simulink model "EMGnodev"  (R2016b)
settings: Solver=FixedStepDiscrete  StartTime=0.0  StopTime=Tfinal  FixedStep=0.01  RelTol=1e-3  EnableMultiTasking=on
settings Model: Creator=philipp  LastModifiedBy=anacsousa
settings DataIOCC: LimitDataPoints=on  SaveFormat=Array
settings OptimizationCC: LifeSpan=Inf
settings DebuggingCC: SolverPrmCheckMsg=warning  MultiTaskRateTransMsg=warning  SFUnexpectedBacktrackingDiag=warning  SFNoUnconditionalDefaultTransitionDiag=warning  SFExecutionAtInitializationDiag=none
settings HardwareCC: ProdBitPerPointer=32  ProdBitPerSizeT=32  ProdBitPerPtrDiffT=32  ProdLargestAtomicFloat=None  ProdIntDivRoundTo=Undefined  ProdEndianess=Unspecified  ProdWordSize=32  ProdHWDeviceType=32-bit Generic
settings ModelReferenceCC: PropagateSignalLabelsOutOfModel=off
settings RTWCC: SystemTargetFile=ert_linux.tlc  MakeCommand=make_rtw OPTS=-DWITH_HW  TemplateMakefile=ert_linux.tmf  Description=Linux Embedded Coder  TargetLang=C++
settings CodeAppCC: IgnoreCustomStorageClasses=off
settings STFCustomTargetCC: ModelReferenceCompliant=off  CombineOutputUpdateFcns=on  ERTCustomFileBanners=on  SupportNonInlinedSFcns=off  RemoveResetFunc=on  SupportVariableSizeSignals=on  MATLABClassNameForMDSCustomization=Simulink.SoftwareTarget.ERTCustomization  GRTInterface=off  SystemTargetFile=ert_linux.tlc
settings ERTTargetCC: ModelReferenceCompliant=off  ParMdlRefBuildCompliant=off  CompOptLevelCompliant=off  ConcurrentExecutionCompliant=off  ERTFirstTimeCompliant=off  SupportContinuousTime=on  SupportVariableSizeSignals=on  ModelStepFunctionPrototypeControlCompliant=off  CPPClassGenCompliant=off  UseToolchainInfoCompliant=off  ExtMode=on  ERTCustomFileTemplate=ert_linux_file_process.tlc  ConvertIfToSwitch=off  SuppressUnreachableDefaultCases=off
settings ConfigComp: CovMetricSettings=dw  CovHtmlReporting=on  CovSaveCumulativeToWorkspaceVar=on  CovSaveSingleToWorkspaceVar=on  CovExternalEMLEnable=off  CovSFcnEnable=off

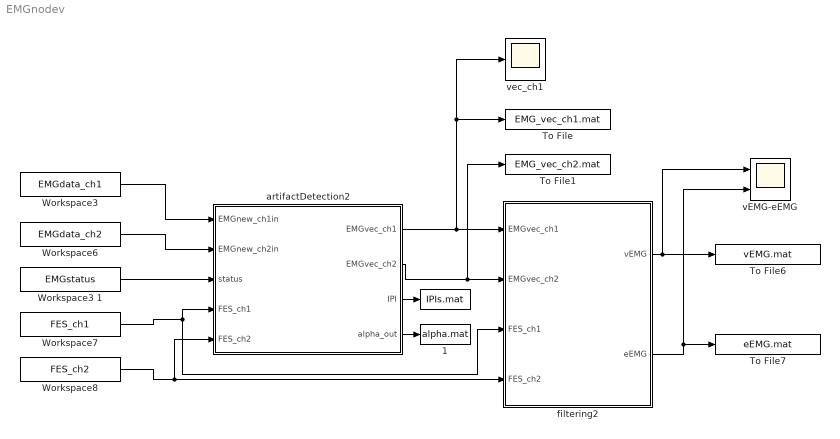
== system EMGnodev ==
  " " : ToFile  Filename=IPIs.mat  MatrixName=IPIs
  " 1" : ToFile  Filename=alpha.mat  MatrixName=alpha
  To File : ToFile  Filename=EMG_vec_ch1.mat  MatrixName=EMG_vec_ch1
  To File1 : ToFile  Filename=EMG_vec_ch2.mat  MatrixName=EMG_vec_ch2
  To File6 : ToFile  Filename=vEMG.mat  MatrixName=vEMG
  To File7 : ToFile  Filename=eEMG.mat  MatrixName=eEMG
  Workspace3 : FromWorkspace  VariableName=EMGdata_ch1  SampleTime=1/25  OutputAfterFinalValue=Holding final value
  Workspace3 1 : FromWorkspace  VariableName=EMGstatus  SampleTime=1/25  OutputAfterFinalValue=Holding final value
  Workspace6 : FromWorkspace  VariableName=EMGdata_ch2  SampleTime=1/25  OutputAfterFinalValue=Holding final value
  Workspace7 : FromWorkspace  VariableName=FES_ch1  SampleTime=1/25  OutputAfterFinalValue=Holding final value
  Workspace8 : FromWorkspace  VariableName=FES_ch2  SampleTime=1/25  OutputAfterFinalValue=Holding final value
  artifactDetection2 : MATLAB Function  TreatAsAtomicUnit=on  mask{emg_f_popup=User-defined, emg_f=1000, stim_f_popup=25, stim_f=25, L=40, peak_popup=Quantiles, complete=on, alpha_auto=on, alpha_init=0.95}
      mask prompts: emg_f_popup "EMG freq [Hz]"; emg_f "Value"; stim_f_popup "Stim freq [Hz]"; stim_f "Value"; peak_popup "Type"; complete "Last complete IPI"; alpha_auto "Automatic alpha"; alpha_init "Initial alpha"
      mask init:
      | alpha_in = [alpha_auto,alpha_init];
      | 
      | 
      | emg_ff = str2double(get_param(gcb,'emg_f'));
      | stim_ff = str2double(get_param(gcb,'stim_f'));
      | L = ceil(emg_f/stim_f);
      | assert(L <= 200, 'Maximum L = emg_f/stim_f is 200.');
  filtering2 : MATLAB Function  TreatAsAtomicUnit=on  mask{emg_f_popup=4000, emg_f=4000, stim_f_popup=25, stim_f=25, Tf=0.04, L=160, emg_ff=4000, stim_ff=25, vol=off, V1=80, V2=155, min_t=0.02, max_t=0.03875, evo=off, E1=10, E2=70, min_te=0.0025, max_te=0.0175, peak_filter=HP filter}
      mask prompts: emg_f_popup "EMG freq [Hz]"; emg_f "Value"; stim_f_popup "Stim freq [Hz]"; stim_f "Value"; Tf "Tf [s]"; L "L [samples]"; vol "Filter volitional"; V1 "Min [samples]"; V2 "Max [samples]"; min_t "Min [s]"; max_t "Max [s]"; evo "Filter evoked"; E1 "Min [samples]"; E2 "Max [samples]"; min_te "Min [s]"; max_te "Max [s]"; peak_filter "Type"
      mask init:
      | % Test L limit
      | emg_ff = str2double(get_param(gcb,'emg_ff'));
      | stim_ff = str2double(get_param(gcb,'stim_ff'));
      | L = ceil(emg_ff/stim_ff);
      | assert(L <= 200, 'Maximum L = emg_f/stim_f is 200.');
      | 
      | % Get V1,V2 and E1,E2 (not checked)
      | maskStr_vol = get_param(gcb,'vol');
      | maskStr_evo = get_param(gcb,'evo');
      | 
      | if ~strcmp(maskStr_vol(2),'n') % check visibility
      |     V1 = 1;    V2 = 1;
      | end  
      | 
      | if ~strcmp(maskStr_evo(2),'n') % check visibility
      |     E1 = 1;    E2 = 1;
      | end
      | 
      | % Test V1,V2,E1,E2 limits
      | assert(V1 >= 1, 'Min_vol must be at least 1.');
      | assert(E1 >= 1, 'Min_evo must be at least 1.');
      | assert(V2 <= L, 'Max_vol must be lower than L.');
      | assert(E2 <= L, 'Max_evo must be lower than L.');
      | 
      | assert(V2 >= 1, 'Max_vol must be at least 1.');
      | assert(E2 >= 1, 'Max_evo must be at least 1.');
      | assert(V1 <= L, 'Min_vol must be lower than L.');
      | assert(E1 <= L, 'Min_evo must be lower than L.');
      | 
      | assert(V2 >= V1, 'Max_vol must be lower than min_vol.');
      | assert(E2 >= E1, 'Max_evo must be lower than min_evo.');
      | 
      | % Create v and e
      | v = [V1;V2];
      | e = [E1;E2];
      | 
      | % init hp filter
      | fc = 50;
      | [z,p,k] = ellip(6,3,50,fc/(emg_ff/2),'high');
      | [B,A] = zp2tf(z,p,k);
      | [F,G,E,D] = tf2ss(B,A);
      | 
      | start_emg = ceil(v(1));
      | stop_emg = ceil(v(2));
      | 
      | N = length(start_emg:stop_emg);
      | Q = eye(N)*D;
      | O = zeros(N,length(E*F));
      | emg_vol = 0;
      | for i = 1:N
      |     for j = i+1:N
      |         Q(j,i) = E*F^(j-i-1)*G;
      |     end
      |     O(i,:)=E*F^(i-1);
      | end
      | 
      | EMGfilter.fc = fc;
      | EMGfilter.Q = Q;
      | EMGfilter.O = O;
      | EMGfilter.start_emg = start_emg;
      | EMGfilter.stop_emg = stop_emg;
  vEMG-eEMG : Scope  NumInputPorts=2
  "vec_ch1 " : Scope
  wires:
  artifactDetection2/1(EMGvec_ch1) -> "vec_ch1 "/1, To File/1, filtering2/1(EMGvec_ch1)
  artifactDetection2/3(IPI) -> " "/1
  filtering2/1(vEMG) -> vEMG-eEMG/1, To File6/1
  filtering2/2(eEMG) -> vEMG-eEMG/2, To File7/1
  Workspace3/1 -> artifactDetection2/1(EMGnew_ch1in)
  Workspace3 1/1 -> artifactDetection2/3(status)
  Workspace7/1 -> filtering2/3(FES_ch1), artifactDetection2/4(FES_ch1)
  Workspace8/1 -> artifactDetection2/5(FES_ch2), filtering2/4(FES_ch2)
  Workspace6/1 -> artifactDetection2/2(EMGnew_ch2in)
  artifactDetection2/2(EMGvec_ch2) -> To File1/1, filtering2/2(EMGvec_ch2)
  artifactDetection2/4(alpha_out) -> " 1"/1

== matlab function EMGnodev/filtering2 ==
  data: EMGvec_ch1 input; EMGvec_ch2 input; vEMG output size=2; eEMG output size=2; FES_ch1 input; FES_ch2 input; peak_filter parameter; EMGfilter parameter; v parameter; e parameter
%% %%%%%%%%%%%%%%%%%%%%%%%%%%%%%%%%%%%%%%%%%%%%%%%%%%%%%%%%%%%%%%%%%%%%%%%%
% block filtering
% by Ana de Sousa (anacsousa@lara.unb.br)
% Last update: Jan 2018
%% %%%%%%%%%%%%%%%%%%%%%%%%%%%%%%%%%%%%%%%%%%%%%%%%%%%%%%%%%%%%%%%%%%%%%%%%
function [vEMG, eEMG] = filtering(EMGvec_ch1,EMGvec_ch2,FES_ch1,FES_ch2,peak_filter,EMGfilter,v,e)

    %% transpose if not column
    if isrow(EMGvec_ch1)
        EMGvec_ch1 = EMGvec_ch1';
    end    
    if isrow(EMGvec_ch2)
        EMGvec_ch2 = EMGvec_ch2';
    end
    
    %% parameters
    stim = or(FES_ch1(1),FES_ch2(1));
    V = zeros(2,1); V(1) = ceil(v(1)); V(2) = ceil(v(2));
    E = zeros(2,1); E(1) = ceil(e(1)); E(2) = ceil(e(2));

    %% choose filter
    switch peak_filter
        %% 'non casual HP filter'
        case 1
            if length(EMGvec_ch1) > 1 % check if it is a vector
                [vEMG_ch1,eEMG_ch1] = noncasualHPfilter(EMGvec_ch1,EMGfilter,stim,V,E);
            else
                vEMG_ch1 = 0; eEMG_ch1 = 0;
            end
            
            if length(EMGvec_ch1) > 1 % check if it is a vector
                [vEMG_ch2,eEMG_ch2] = noncasualHPfilter(EMGvec_ch2,EMGfilter,stim,V,E);
            else
                vEMG_ch2 = 0; eEMG_ch2 = 0;                
            end            
        %% 'lambda and gama filters' 
        case 2       
            if length(EMGvec_ch1) > 1 % check if it is a vector
                [vEMG_ch1,eEMG_ch1] = lambdafilter(EMGvec_ch1,stim,V,E);
            else
                vEMG_ch1 = 0; eEMG_ch1 = 0;
            end
            if length(EMGvec_ch1) > 1 % check if it is a vector
                [vEMG_ch2,eEMG_ch2] = lambdafilter(EMGvec_ch2,stim,V,E);  
            else
                vEMG_ch2 = 0; eEMG_ch2 = 0;                
            end       
        otherwise % 'otherwise'
            error('No filter was selected.');
    end
    
    % extract some information from vector
    vEMG = [mean(abs(vEMG_ch1),'omitnan');mean(abs(vEMG_ch2),'omitnan')];
    eEMG = [mean(abs(eEMG_ch1),'omitnan');mean(abs(eEMG_ch2),'omitnan')]; 
end

%% noncasualHPfilter %%%%%%%%%%%%%%%%%%%%%%%%%%%%%%%%%%%%%%%%%%%%%%%%%%%%%%
function [vEMG,eEMG] = noncasualHPfilter(EMG,EMGfilter,stim,V,E)
   
    %% extract EMGv [V1:V2] 
    V1 = V(1);            V2 = V(2);
    EMG_V = bound_emg(V2 - V1 + 1);
    for i = 1:V2 - V1 + 1
        EMG_V(i) = EMG(V1 + i);
    end
%     too_large = 10e25;
            
    %% get vol
    % filter parameters    
    Q = EMGfilter.Q;
    O = EMGfilter.O;
    QQ = Q'*Q;
    R_O = fliplr(O);
%     if norm(diff(EMG_V),2)>too_large
%         disp('norm too large: possible spike');
%     end
    % if its in condition to be filtered
    
    emg_v_median = quantile(abs(EMG_V),0.5);
    is_no_trash =  (max(abs(EMG_V))<100*emg_v_median);
   
    if ((sum(EMG_V)~=0)&&is_no_trash)
      
        % remove mean
        EMG_V = EMG_V - mean(EMG_V,'omitnan');

        % HP filter
        EMG_V(isnan(EMG_V)) = 1;
        x_init_opt = ([Q'*O R_O]'*[Q'*O R_O])'\((-Q'*Q*EMG_V)'*[Q'*O R_O])';
        EMG_HP = QQ*EMG_V + [Q'*O R_O]*x_init_opt;

        vEMG = EMG_HP;
    else
        vEMG = bound_emg(V2 - V1 + 1);
    end
            
%     if mean(abs(vEMG),'omitnan')>50000
%         disp();        
%     end
    %% get evoked
    if stim
        % extract EMGe [E1:E2]
        E1 = E(1);            E2 = E(2);
        EMG_E = bound_emg(E2 - E1 + 1);
        for i = 1:E2 - E1 + 1
            EMG_E(i) = EMG(E1 + i);
        end
        
        % remove mean
        EMG_E = EMG_E - mean(EMG_E,'omitnan');
        
        EMG_E(isnan(EMG_E)) = 1;
        % mav
        mav = sum(abs(EMG_E));

        eEMG = mav*bound_emg2(E2 - E1 + 1);
    else
        eEMG = bound_emg(V2 - V1 + 1);        
    end    
end

%% lambdafilter %%%%%%%%%%%%%%%%%%%%%%%%%%%%%%%%%%%%%%%%%%%%%%%%%%%%%%
function [vEMG, eEMG] = lambdafilter(EMG,stim,V,E)
    
    %% extract vEMG [V1:V2]
    V1 = V(1);    V2 = V(2);
    buffer_vol = V2 - V1;
    EMG_V = EMG(V1:V2-1);
    EMG_V(isnan(EMG_V)) = 1;
    
    %% extract eEMG [E1:E2]
    E1 = E(1); E2 = E(2);
    buffer_evoked = E2 - E1;
    EMG_E = EMG(E1:E2-1);
    EMG_E(isnan(EMG_E)) = 1;
    
    %% make buffers
    persistent  MwavesDelayedVol; 
    if isempty(MwavesDelayedVol)
        MwavesDelayedVol = MwavesDelayed_bound(buffer_vol);
    end
    
    persistent  MwavesDelayedEvoked; 
    if isempty(MwavesDelayedEvoked)
        MwavesDelayedEvoked = MwavesDelayed_bound(buffer_evoked);
    end

    %% VOL
    X = MwavesDelayedVol';
    Y = EMG_V;    
    TH = X\Y;
    MWhat = TH'*X';
    
    EMG_Ve = EMG_V'-MWhat;

    % get gama    
    gama = norm(EMG_Ve); % scaled 1-norm of the vector
    vEMG = ones(size(MWhat'))*gama; % return
    
    % update vol buffer
    for i = 0:4 
        MwavesDelayedVol(6-i,1:buffer_vol) = MwavesDelayedVol(6-i-1,1:buffer_vol);
    end
    MwavesDelayedVol(1,1:buffer_vol) = EMG_V;

    %% EVOKED        
    if stim
        X = MwavesDelayedEvoked';
        Y = EMG_E;    
        TH = X\Y;
        MWhat = TH'*X';

        % get lambda
        lambda = norm(MWhat); % scaled 1-norm of the vector
        eEMG = ones(size(MWhat'))*lambda; % return
         
        % update evoked buffer
        for i = 0:4 
            MwavesDelayedEvoked(6-i,1:buffer_evoked) = MwavesDelayedEvoked(6-i-1,1:buffer_evoked);
        end
        MwavesDelayedEvoked(1,1:buffer_evoked) = EMG_E;
    else
        eEMG = zeros(size(MWhat'));
    end

end

%% Specify Upper Bounds for Local Variables
% see more: (https://de.mathworks.com/help/simulink/ug/variable-size-data-when-dynamic-memory-allocation-is-disabled.html)
function y = bound_emg(n) %#last_emg_vec
    % f_emg_max/f_stim_max <--- maybe this can change
    assert(n <= 200, 'Buffer size is higher than 200.'); 
    y = zeros(n,1);
end
function y = bound_emg2(n) %#last_emg_vec
    % f_emg_max/f_stim_max <--- maybe this can change
    assert(n <= 200, 'Buffer size is higher than 200.'); 
    y = ones(n,1);
end
function y = MwavesDelayed_bound(n) %#past_emg_vec
    % f_emg_max/f_stim_max * size of buffer <--- maybe this can change
    assert(n <= 2048/10*6, 'Bounds for past_emg_vec are higher than it should be.'); 
    y = zeros(6,n);
end

== matlab function EMGnodev/artifactDetection2 ==
  data: EMGnew_ch1in input; EMGnew_ch2in input; EMGvec_ch1 output size=200; status input; FES_ch1 input; FES_ch2 input; peak_popup parameter; EMGvec_ch2 output size=200; L parameter; complete parameter size=1; IPI output size=1; alpha_in parameter size=2; alpha_out output
%% %%%%%%%%%%%%%%%%%%%%%%%%%%%%%%%%%%%%%%%%%%%%%%%%%%%%%%%%%%%%%%%%%%%%%%%%
% block artifactDetection
% by Ana de Sousa (anacsousa@lara.unb.br)
% Last update: Feb-2018
%% %%%%%%%%%%%%%%%%%%%%%%%%%%%%%%%%%%%%%%%%%%%%%%%%%%%%%%%%%%%%%%%%%%%%%%%%

function [EMGvec_ch1, EMGvec_ch2, IPI, alpha_out]   = artifactDetection(EMGnew_ch1in, EMGnew_ch2in, status, FES_ch1, FES_ch2, peak_popup, L, complete, alpha_in)

    %% transpose if not column
    if isrow(EMGnew_ch1in)
        EMGnew_ch1 = EMGnew_ch1in';
    else
        EMGnew_ch1 = EMGnew_ch1in;
    end    
    if isrow(EMGnew_ch2in)
        EMGnew_ch2 = EMGnew_ch2in';
    else
        EMGnew_ch2 = EMGnew_ch2in;
    end

    %% Definition of parameters  
    b = 3.1;
    buffer_size = ceil(L*b);
    buffer_offsets_size = 5;
    n_stims = floor(b)+1;   
    ch_conn = [0,0];
    
    %% Step 0: pre-check (Verification of connected channels)
    if EMGnew_ch1 == 0
        ch_conn(1) = 0;
    else
        ch_conn(1) = 1;
    end
    
    if EMGnew_ch2 == 0
        ch_conn(2) = 0;
    else
        ch_conn(2) = 1;
    end
    
    %% Step 1: create and update buffers
    persistent  emg_buffer; 
    if isempty(emg_buffer)
        emg_buffer = bound_buffer2(buffer_size);
    end
    
    persistent  buffer_offsets_ch1;
    if isempty(buffer_offsets_ch1) 
        buffer_offsets_ch1 = bound_buffer(buffer_offsets_size);
    end
    
    persistent  buffer_offsets_ch2;
    if isempty(buffer_offsets_ch2) 
        buffer_offsets_ch2 = bound_buffer(buffer_offsets_size);
    end
    
    persistent  last_stim; 
    if isempty(last_stim)
        last_stim = bound_stim(n_stims);
    end
    
    %% alpha definitions
    persistent  alpha;
    if isempty(alpha) 
        alpha = alpha_in(2); % init alpha with second value
    end
    
    % Updates buffer from EMG data
    EMGstatus = int16(status(1));
    
    if (EMGstatus >= 1)   % ch1
        if EMGstatus > buffer_size % limit EMGstatus size to avoid errors if incorrect freq is put
            EMGstatus = int16(buffer_size);
            disp('Warning: status > buffer size, check EMG and stimulation frequencies.');
        end
        if size(EMGnew_ch1,1) > 1
            emg_buffer(1:buffer_size,1) = [emg_buffer(EMGstatus+1:buffer_size,1);EMGnew_ch1(1:EMGstatus)];
        end
    end
    
    if (EMGstatus >= 1)   % ch2
        if size(EMGnew_ch2,1) > 1
            emg_buffer(1:buffer_size,2) = [emg_buffer(EMGstatus+1:buffer_size,2);EMGnew_ch2(1:EMGstatus)];
        end
    end
    
    % Updates buffer from FES data
    stim = or(FES_ch1(1),FES_ch2(1));    
    last_stim(1:n_stims) = [last_stim(2:n_stims);stim];
    idx = last_stim ~= 0; 
    n_stims = sum(idx(:)); % # of artifacts expected, relates to buff_size;
        
    %% Step 2: artifacts detection (all artifacts found)
    IPI_c = buffer_size - L;
    IPI_i = buffer_size - L;
    
    % considers if channels are conn and stimulated 
    if (ch_conn(1)==1)||(ch_conn(2)==1) 
        if n_stims % if there is any pulse
            
            if (~isequal(last_stim,[0;0;0;1]))&&(~isequal(last_stim,[1;0;0;0])) % transitions of stim
                % find all points
                [all_pts] = choose_algorithm(peak_popup,alpha,emg_buffer);
                
                    %% consider # clusters vs alpha 
                    n_clusters = count_clusters(all_pts,L);
                    
                    %% if automatic alpha was chosen:
                    if alpha_in(1)
                        n_exp_pulses = 3;                        
                        d_alpha = n_clusters - n_exp_pulses;
                        
                        % if found pulses are different from expected pulses
                        if ~((n_clusters == 3) || (n_clusters == 4) || (n_clusters == 5))
                            % alpha limits
                            switch peak_popup
                                case 1 % 'var'
                                    ss = 0.1;
                                    alpha = alpha*(1+sign(d_alpha)*ss);
                                    
                                    if alpha < 10^-3
                                        alpha = 10^-3;
                                    elseif alpha > 5
                                        alpha = 5;
                                    end
                                    
                                case 2 % 'MAD'  
                                    ss = 0.1;
                                    alpha = alpha*(1+sign(d_alpha)*ss);
                                    
                                    if alpha < 2
                                        alpha = 2;
                                    elseif alpha > 5000
                                        alpha = 5000;
                                    end
                                case 3 % 'q'   
                                    ss = 0.01;
                                    alpha = alpha*(1+sign(d_alpha)*ss);
                                    
                                    if alpha < 0.9 %% simulink does not understand that we already bounded it...
                                        alpha = 0.9;
                                    elseif alpha >  0.985
                                        alpha = 0.985;
                                    end
                                otherwise % 'otherwise'
                                    error('No algorithm was selected.');
                            end   
                        end
                    end

                %% Step 3: determine IPI based on found artifacts
                [IPI_c,IPI_i] = cluster_peaks(all_pts, L, last_stim, n_stims);
            end
        end
    end
    
    %% Step 4: extract last full emg period
    if complete % return IPI complete or incomplete
        IPI = IPI_c;        
        % check if enough samples  
        if (IPI(1) < 0 )||(IPI(1) > buffer_size - L) 
            IPI(1) = buffer_size - L;
        end
    else
        IPI = IPI_i;
    end
    
    [ EMGvec_ch1, buffer_offsets_ch1 ] = extractLastFullEMG(IPI, emg_buffer(:,1), buffer_offsets_ch1, L, complete); 
    [ EMGvec_ch2, buffer_offsets_ch2 ] = extractLastFullEMG(IPI, emg_buffer(:,2), buffer_offsets_ch2, L, complete);
    
    alpha_out = alpha;
end

%% %%%%%%%%%%%%%%%%%%%%%%%%%%%%%%%%%%%%%%%%%%%%%%%%%%%%%%%%%%%%%%%%%%%%%%%%%
%% %%%%%%%%%%%%%%%%%%%%%%%%%%%%%%%%%%%%%%%%%%%%%%%%%%%%%%%%%%%%%%%%%%%%%%%%%
%% %%%%%%%%%%%%%%%%%%%%%%%%%%%%%%%%%%%%%%%%%%%%%%%%%%%%%%%%%%%%%%%%%%%%%%%%%

%% Specify Upper Bounds for Local Variables
% see more: (https://de.mathworks.com/help/simulink/ug/variable-size-data-when-dynamic-memory-allocation-is-disabled.html)
function y = bound_buffer(n)
    assert(n <= 5*4000/10, 'Buffer size is higher than 2000.'); 
    y = zeros(n,1);
end

function y = bound_buffer2(n)
    assert(n <= 5*4000/10, 'Buffer size is higher than 2000.');
    y = zeros(n,2);
end

function y = bound_stim(n)
    assert(n <= 10, 'Number of stims is higher than 10. '); 
    y = zeros(n,1);
end

function y = bound_vec(n)
    assert(n <= 5*4000/10, 'Buffer size is higher than 2000.'); 
    y = zeros(1,n);
end

%% Choose the algorithm to find all peaks %%%%%%%%%%%%%%%%%%%%%%%%%%%%%%%%%
function [all_IPI] = choose_algorithm(peak_popup,alpha,emg_vec)
    n_loc_found = length(emg_vec);
    all_IPI = zeros(1,n_loc_found);
    
    switch peak_popup
        case 1 % 'std'            
            DE1 = (diff(diff(emg_vec(:,1))));
            DE2 = (diff(diff(emg_vec(:,2))));
            mean_d1 = mean(DE1,'omitnan');  mean_d2 = mean(DE2,'omitnan');
            std_d1 = std(DE1,'omitnan');    std_d2 = std(DE2,'omitnan');
            
            % look for points
            k_max1 = mean_d1+std_d1*alpha;  k_max2 = mean_d2+std_d2*alpha;
            k_min1 = mean_d1-std_d1*alpha;  k_min2 = mean_d2-std_d2*alpha;
            
            loc_found1 = find(DE1 > k_max1 | DE1 < k_min1); %find std1
            loc_found2 = find(DE2 > k_max2 | DE2 < k_min2); %find std2
            loc_found = union(loc_found1,loc_found2);

        case 2 % 'MAD'
            DE1 = (diff(diff(emg_vec(:,1))));
            DE2 = (diff(diff(emg_vec(:,2))));
            mean_d1 = median(DE1,'omitnan');  mean_d2 = median(DE2,'omitnan');
            mad_d1 = mad(DE1,1);            mad_d2 = mad(DE2,1);
            
            % look for points
            k_max1 = mean_d1+mad_d1*alpha;  k_max2 = mean_d2+mad_d2*alpha;
            k_min1 = mean_d1-mad_d1*alpha;  k_min2 = mean_d2-mad_d2*alpha;
            
            loc_found1 = find(DE1 > k_max1 | DE1 < k_min1); %find std1
            loc_found2 = find(DE2 > k_max2 | DE2 < k_min2); %find std2
            loc_found = union(loc_found1,loc_found2);
            
        case 3 % 'quantiles'
            DE1 = (diff(diff(emg_vec(:,1))));
            DE2 = (diff(diff(emg_vec(:,2))));
            
            
            if alpha < 0.9 %% simulink does not understand that we already bounded it...
                alpha = 0.9;
            elseif alpha >  0.985
                alpha = 0.985;
            end

            q_max1 = quantile(DE1,alpha);
            q_min1 = quantile(DE1,1-alpha);
            q_max2 = quantile(DE2,alpha); 
            q_min2 = quantile(DE2,1-alpha);
            loc_found1 = find( DE1>q_max1(1) | DE1<q_min1(1)) ; %find quantiles DE1
            loc_found2 = find( DE2>q_max2(1) | DE2<q_min2(1)) ; %find quantiles DE2
            loc_found = union(loc_found1,loc_found2);   
            
        otherwise % 'otherwise'
            error('No algorithm was selected.');
    end
    
    % Adjust vector to return
    if ~isempty(loc_found)
        a = min(n_loc_found,length(loc_found));  %check which is smaller

        for i=1:a % do not extrapolate the vector
            all_IPI(i) = loc_found(i);
        end
    end  
end

%% Extract last full emg period from last IPI %%%%%%%%%%%%%%%%%%%%%%%%%%%%%
function [ EMGvec, offsets_buffer ] = extractLastFullEMG(IPI, emg_buffer, offsets_buffer, L, complete)

	% Parameters
    EMGvec = NaN(1,200);
    buffer_size = length(emg_buffer);
    buffer_size_offsets = length(offsets_buffer); 
    
    %% update the emg vec with the new COMPLETE peak (until L)
    
    %% if IPI is not zero, we return position based on IPI (complete or incomplete)
    if IPI(1) ~= 0
        %% now we consider if it is complete or incomplete
        if complete %% complete
            for i = 1:L 
                EMGvec(i) = emg_buffer(IPI + i);
            end
        else %% incomplete
            %% if there is enough samples, just fill (buffer_size-L)
            if IPI(1) <= buffer_size - L
                for i = 1:L 
                    EMGvec(i) = emg_buffer(IPI + i);
                end
            %% if there is not, fill until possible (buffer_size-IPI)
            else
                for i = 1:buffer_size-IPI 
                    EMGvec(i) = emg_buffer(IPI + i);
                end
            end
        end
    %% otherwise, something went wrong before, so return EMGvec as zero
    else
        for i = 1:L 
            EMGvec(i) = 0;
        end
    end
        
    %% Remove offset
    for i = 1:buffer_size_offsets-1
        offsets_buffer(end-i+1) = offsets_buffer(end-i);
    end
    x = 0;
    c = buffer_size_offsets;
    for i = 1:buffer_size_offsets
        x = x + emg_buffer(ceil(0.8*L) + i);
    end
    offsets_buffer(1) = x/c; %mean

    EMGvec = EMGvec - mean(offsets_buffer);
    EMGvec = EMGvec.'; % return
end


%% Cluster peaks %%%%%%%%%%%%%%%%%%%%%%%%%%%%%%%%%%%%%%%%%%%%%%%%%%%%%%%%%%%
function [IPI_c,IPI_i] = cluster_peaks(all_pts, L, last_stim, n_stims)

    %% parameters
    buffer_size = length(all_pts);
    if ~(last_stim(end) == 0) %adjust # of expected stims
        n_stims = n_stims-1;
    end
    
    %% find clusters and count # of elements in each cluster
    ind_del = all_pts == 0;    points = all_pts;
    points(ind_del) = [];
    changes = find((diff(points) > L*0.1))+1; % find where cluster change
    n_clusters = length(changes) + 1; % # of clusters found
    
    a = zeros(1,n_clusters);
    b = zeros(1,n_clusters);
    
    if(n_clusters > 1) % more than one cluster found
        u = [changes(1)-1, diff(changes), length(points) - changes(end) + 1];        
        % saving first (a) and last (b) points of each cluster (i)
        for i=1:n_clusters
            if i == 1
                a(i) = points(1);
                b(i) = points(changes(i)-1);
            elseif i == n_clusters
                a(i) = points(changes(i-1));
                b(i) = points(end);
            else
                a(i) = points(changes(i-1));
                b(i) = points(changes(i)-1);
            end
        end
    else % only one (or none) cluster found
        u = length(points);
        if ~isempty(points)
            a = points(1);
            b = points(end);
        else
            a = 1;
            b = 1;
        end
    end
        
    %% create base and real vectors
    vec_base = bound_vec(buffer_size);    
    vec_real = bound_vec(buffer_size);
    
    if floor(mean(u)) % base
        if mean(b-a)+1 < ceil(L/2) % limit number of points
            n_pts = ceil(mean(b-a)+1);
        else
            n_pts = ceil(L/2);
        end
    else 
        n_pts = 5;
    end
    
    init = 1;    
    for i = 1:n_stims %vec_base
        vec_base((init + (i-1)*L):init + n_pts + (i-1)*L - 1) = 1;
    end
    
    for i = 1:length(a) %vec_real
        vec_real(a(i)) = 1;
        for j = 1:b(i)-a(i)
            vec_real(a(i)+j) = 1;
        end
    end
    
    %% Correlate vec_base and vec_real to shift them
    [acor,lag] = xcorr(vec_base', vec_real');
    [~,I] = max(abs(acor));
    lagDiff = abs(lag(I));
            
    %% Transition state (#stims = 1), IPI = lagDiff
    % Everthing bellow considers the transitions between on and off stim:
    %   . When the charge shifts on -> off, or off -> on, the stimulator
    %   needs a period to respond in real time.
    %   . Also we need to consider if we want a complete or an incomplete
    %   IPI.
    IPI_c = buffer_size - L;
    IPI_i = buffer_size - L;
    
    % TRANSITIONS
    adjust_diff = 0;
    if isequal(last_stim,[0;0;1;1]) % transition off->on (for IPI_i)
        IPI_i = lagDiff+adjust_diff;
        IPI_c = 0;
    elseif isequal(last_stim,[1;1;0;0]) % transition on->off (for IPI_c)
        new_pos = find( points > 0.95*(lagDiff+L+adjust_diff) ); % look for the 1st pulse after
        if new_pos
            IPI_c = points(new_pos(1))+adjust_diff;
        end
    elseif isequal(last_stim,[0;1;1;1]) % transition off->on (for in and complete)
        IPI_c = lagDiff+2;
        new_pos = find( points > 0.95*(lagDiff+L+adjust_diff) ); % look for next pulse
        if new_pos
            IPI_i = points(new_pos(1))+adjust_diff;
        end
    % STABLE
    else  
        new_pos = find( points > 0.95*(lagDiff+L+adjust_diff) ); % look for the 1st pulse after
        if new_pos
            IPI_c = points(new_pos(1))+adjust_diff;
        end

        new_pos2 = find( points > 0.95*(lagDiff+2*L+adjust_diff) ); % look for the 2nd pulse after
        if new_pos2
            IPI_i = points(new_pos2(1))+adjust_diff;
        end
    end
end

%% Count number of clusters %%%%%%%%%%%%%%%%%%%%%%%%%%%%%%%%%%%%%%%%%%%%%%%%
function n_clusters = count_clusters(all_pts,L)
    % make a vector without the zeros
    ind_del = all_pts == 0;     points = all_pts;
    points(ind_del) = [];  
    
    % count clusters considering a min diff between points
    changes = find((diff(points) > L*0.1))+1;
    n_clusters = length(changes) + 1;
end
